simulink model "master_slave_ejemplo_propio"  (R2018a)
settings: Solver=ode45  StartTime=0.0  StopTime=20  MaxStep=1e-2  RelTol=1e-3
InitFcn:
  | ejemplo_2
values from neighbouring files (symbols this model uses):
  ki = kt(1,3)    [control_nolineal_linealizacion_entrada_estado.m]    (also in e_mimo.m; ej_mimo.m = kt(:,2+1:end); ej_mimo2.m = kt(:,2+1:end); ejemplo_2.m)
  kp = kt(1,1:2)    [control_nolineal_linealizacion_entrada_estado.m]    (also in e_mimo.m; ej_mimo.m = kt(:,1:2); ej_mimo2.m = kt(:,1:2); ejemplo_2.m)
libraries: simulink x1
settings Model: Creator=carma  LastModifiedBy=carma

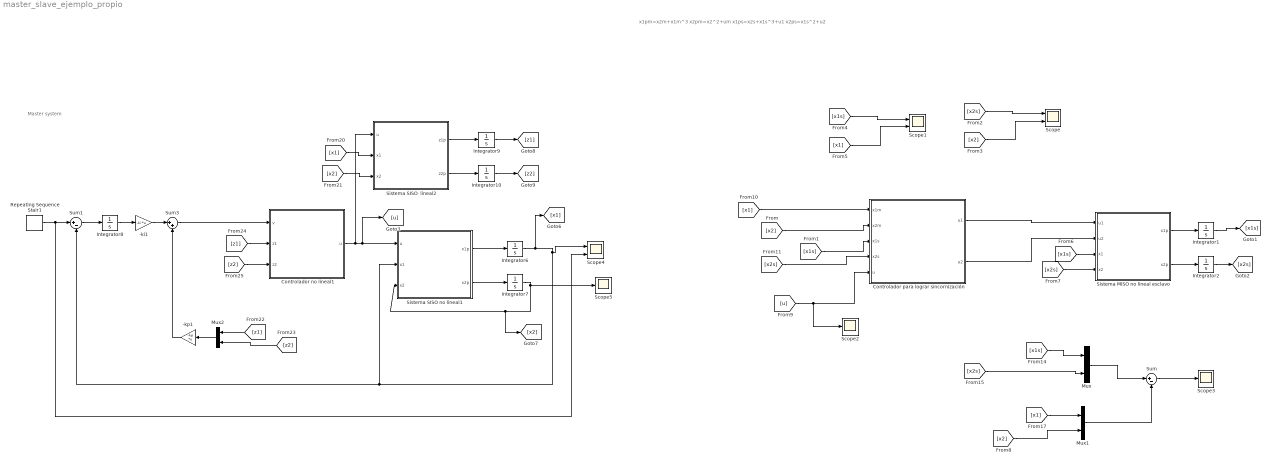
== system master_slave_ejemplo_propio ==
  note: Master system
  note: x1pm=x2m+x1m^3
      | x2pm=x2^2+um
      |
      | x1ps=x2s+x1s^3+u1
      | x2ps=x1s^2+u2
  -ki1 : Gain  Gain=-ki  Multiplication=Matrix(K*u) (u vector)
  -kp1 : Gain  Gain=-kp  Multiplication=Matrix(K*u) (u vector)
  Controlador no lineal1 : MATLAB Function  TreatAsAtomicUnit=on
  Controlador para lograr sincornización : MATLAB Function  TreatAsAtomicUnit=on
  Integrator{1..2,6..10} (7 alike) : Integrator
  Mux : Mux  Inputs=2
  Mux1 : Mux  Inputs=2
  Mux2 : Mux  Inputs=2
  Repeating Sequence Stair1 : simulink/Sources/Repeating Sequence Stair  OutValues=[0.5 0.4 -0.2 0.1 0.3].'  tsamp=2  OutMin=[]  OutMax=[]  OutDataTypeStr=double  OutputDataTypeScalingMode=double  OutDataType=fixdt(0,8)  ConRadixGroup=Best Precision: Vector-wise  OutScaling=2^-12
  Scope : Scope  NumInputPorts=2
  Scope1 : Scope  NumInputPorts=2
  Scope2 : Scope
  Scope3 : Scope
  Scope4 : Scope  NumInputPorts=2
  Scope5 : Scope
  Sistema MISO no lineal esclavo : MATLAB Function  TreatAsAtomicUnit=on
  Sistema SISO  lineal2 : MATLAB Function  TreatAsAtomicUnit=on
  Sistema SISO no lineal1 : MATLAB Function  TreatAsAtomicUnit=on
  Sum : Sum  Inputs=|+-
  Sum1 : Sum  Inputs=|+-
  Sum3 : Sum  Inputs=|++
  wires:
  [x2] -> Controlador para lograr sincornización/2(x2m)
  [x1s] -> Controlador para lograr sincornización/3(x1s)
  [x2s] -> Scope/1
  [x2] -> Scope/2
  [x1] -> Scope1/2
  [x1s] -> Scope1/1
  [x1] -> Controlador para lograr sincornización/1(x1m)
  [x2s] -> Controlador para lograr sincornización/4(x2s)
  Mux1/1 -> Sum/2
  [x1] -> Mux1/1
  [x1s] -> Mux/1
  Mux/1 -> Sum/1
  [x2s] -> Mux/2
  Sum/1 -> Scope3/1
  Sum1/1 -> Integrator8/1
  Sistema SISO no lineal1/2(x2p) -> Integrator7/1
  Sum3/1 -> Controlador no lineal1/1(v)
  Sistema SISO  lineal2/1(z1p) -> Integrator9/1
  [z1] -> Mux2/1
  Controlador no lineal1/1(u) -> Sistema SISO  lineal2/1(u), [u], Sistema SISO no lineal1/1(u)
  Integrator9/1 -> [z1]
  -ki1/1 -> Sum3/1
  Sistema SISO  lineal2/2(z2p) -> Integrator10/1
  Sistema SISO no lineal1/1(x1p) -> Integrator6/1
  Integrator7/1 -> Scope5/1, [x2], Sistema SISO no lineal1/3(x2)
  [x1] -> Sistema SISO  lineal2/2(x1)
  Integrator8/1 -> -ki1/1
  [x2] -> Sistema SISO  lineal2/3(x2)
  Mux2/1 -> -kp1/1
  Integrator6/1 -> [x1], Scope4/1, Sum1/2, Sistema SISO no lineal1/2(x1)
  [z2] -> Controlador no lineal1/3(z2)
  -kp1/1 -> Sum3/2
  Integrator10/1 -> [z2]
  [z1] -> Controlador no lineal1/2(z1)
  Repeating Sequence Stair1/1 -> Scope4/2, Sum1/1
  [z2] -> Mux2/2
  Controlador para lograr sincornización/1(u1) -> Sistema MISO no lineal esclavo/1(u1)
  Controlador para lograr sincornización/2(u2) -> Sistema MISO no lineal esclavo/2(u2)
  Sistema MISO no lineal esclavo/1(x1p) -> Integrator1/1
  Sistema MISO no lineal esclavo/2(x2p) -> Integrator2/1
  Integrator1/1 -> [x1s]
  Integrator2/1 -> [x2s]
  [x1s] -> Sistema MISO no lineal esclavo/3(x1)
  [x2s] -> Sistema MISO no lineal esclavo/4(x2)
  [x2] -> Mux1/2
  [u] -> Scope2/1, Controlador para lograr sincornización/5(u)

== matlab function master_slave_ejemplo_propio/Sistema MISO no lineal esclavo ==
  data: u1 input; u2 input; x1 input; x2 input; x1p output; x2p output
function [x1p,x2p]= fcn(u1,u2,x1,x2)




x1p=x2+x1^3+u1;
x2p=x1^2+u2;

== matlab function master_slave_ejemplo_propio/Controlador para lograr sincornización ==
  data: x1m input; u1 output; x2m input; x1s input; x2s input; u2 output; u input
function [u1,u2] = fcn(x1m,x2m,x1s,x2s,u)




%ex1=x1s-x1m;
ex2=x2s-x2m;

k12=1;
k22=-1;

v1=-k12*ex2
v2=-k22*ex2;

u1=v1;
u2=v2+x1m^2-x1s^2+u;

== matlab function master_slave_ejemplo_propio/Controlador no lineal1 ==
  data: v input; u output; z1 input; z2 input
function u = fcn(v,z1,z2)

%parametros
a=4;


u=-3*z1^2*z2-z1^2+v

%s=5;
%syms y
%Cx3=(2+10^(pk2-y))/(1+10^(pk2-y)+10^(pk1+pk2-2*y));
%h=-x1+x2-x3*Cx3+10^(-y)-10^(y-pkw)==0;

%s=double(solve(h));

== matlab function master_slave_ejemplo_propio/Sistema SISO  lineal2 ==
  data: u input; z1p output; x1 input; x2 input; z2p output
function [z1p,z2p]= fcn(u,x1,x2)

z1p=x2+x1^3;
z2p=u+x1^2+3*x1^2*(x2+x1^3);


% z1p=z2;
% z2p=v;

%s=5;
%syms y
%Cx3=(2+10^(pk2-y))/(1+10^(pk2-y)+10^(pk1+pk2-2*y));
%h=-x1+x2-x3*Cx3+10^(-y)-10^(y-pkw)==0;

%s=double(solve(h));

== matlab function master_slave_ejemplo_propio/Sistema SISO no lineal1 ==
  data: u input; x1p output; x1 input; x2 input; x2p output
function [x1p,x2p]= fcn(u,x1,x2)

%parametros
a=4;



x1p=x2+x1^3
x2p=x1^2+u;

%s=5;
%syms y
%Cx3=(2+10^(pk2-y))/(1+10^(pk2-y)+10^(pk1+pk2-2*y));
%h=-x1+x2-x3*Cx3+10^(-y)-10^(y-pkw)==0;

%s=double(solve(h));
